simulink model "Model_v2"  (R2016b)
settings: Solver=VariableStepAuto  StartTime=0.0  StopTime=2  MaxStep=0.01  RelTol=1e-3
InitFcn:
  | start
values from neighbouring files (symbols this model uses):
  A = [0 0 1 ... (first row only)    [matrix_set.m]
  B = [0 ... (first row only)    [matrix_set.m]
  K = lqr(A,B,QQ,RR)    [matrix_set.m]
  Psi0 = pi/12    (= 0.261799387799)    [start_config.m]
  Psi_d0 = 0    [start_config.m]
  R = 0.0275    [variables_set.m]
  Theta_d0 = 0    [start_config.m]
  Umax = 8.2    [variables_set.m]
libraries: vrlib x4, simulink_extras x3
settings Model: PauseTimes=1  SnapshotBufferSize=8000  Creator=danii  LastModifiedBy=danii
settings SolverCC: ZeroCrossAlgorithm=Adaptive
settings ConfigComp: PSAutoStubLUT=on

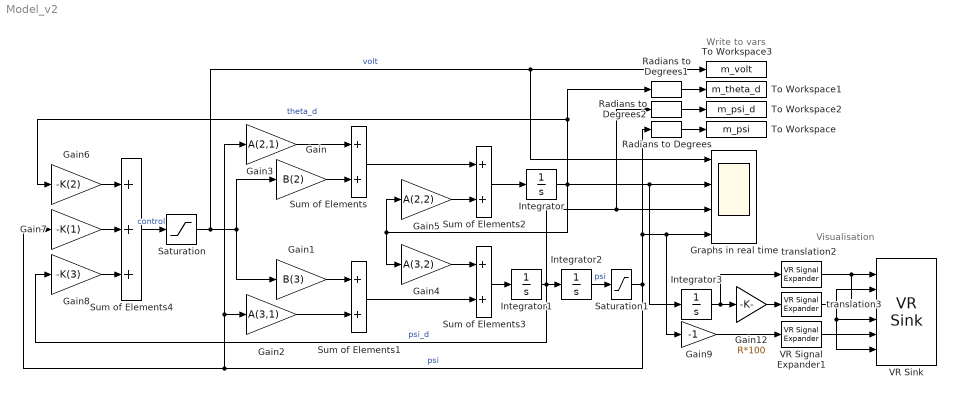
== system Model_v2 ==
  note: Visualisation
  note: Write to vars
  Gain : Gain  Gain=B(2)
  Gain1 : Gain  Gain=B(3)
  Gain12 : Gain  Gain=R*100
  Gain2 : Gain  Gain=A(3,1)
  Gain3 : Gain  Gain=A(2,1)
  Gain4 : Gain  Gain=A(3,2)
  Gain5 : Gain  Gain=A(2,2)
  Gain6 : Gain  Gain=-K(2)
  Gain7 : Gain  Gain=-K(1)
  Gain8 : Gain  Gain=-K(3)
  Gain9 : Gain  Gain=-1
  Graphs in real time : Scope  NumInputPorts=4
  Integrator : Integrator  InitialCondition=Theta_d0
  Integrator1 : Integrator  InitialCondition=Psi_d0
  Integrator2 : Integrator  InitialCondition=Psi0
  Integrator3 : Integrator  InitialCondition=Theta_d0
  Radians to Degrees : simulink_extras/Transformations/Radians to Degrees
  Radians to Degrees1 : simulink_extras/Transformations/Radians to Degrees
  Radians to Degrees2 : simulink_extras/Transformations/Radians to Degrees
  Saturation : Saturate  UpperLimit=Umax  LowerLimit=-Umax
  Saturation1 : Saturate  UpperLimit=pi/180*95  LowerLimit=-pi/180*95
  Sum of Elements{,1..3} (4 alike) : Sum  Inputs=2
  Sum of Elements4 : Sum  Inputs=3
  To Workspace : ToWorkspace  VariableName=m_psi  SampleTime=-1
  To Workspace1 : ToWorkspace  VariableName=m_theta_d  SampleTime=-1
  To Workspace2 : ToWorkspace  VariableName=m_psi_d  SampleTime=-1
  To Workspace3 : ToWorkspace  VariableName=m_volt  SampleTime=-1
  VR Signal Expander1 : vrlib/VR Signal Expander  outwidth=4  outidx=[4]
  VR Sink : vrlib/VR Sink  InstantiateOnLoad=on  SampleTime=0.005  ViewEnable=on  RemoteChange=off  RemoteView=off  FieldsWritten=wheel_1.rotation.4.1.1.double#wheel_1.translation.3.1.1.double#wheel_2.rotation.4.1.1.double#wheel_2.translation.3.1.1.double#body.rotation.4.1.1.double#body.translation.3.1.1.double  WorldFileName=Model.wrl  AutoView=off  VideoDimensions=[]  AllowVariableSize=off  FigureProperties="{'Position', 'Name', 'Viewpoint', 'CameraBound', 'CameraDirection', 'CameraPosition', 'CameraUpVector', 'ZoomFactor', 'Antialiasing', 'Headlight', 'Lighting', 'NavPanel', 'Sound', 'StatusBar', 'Stereo3D', 'Stereo3DCameraOffset', 'Stereo3DHIT', 'ToolBar', 'Textures', 'Transparency', 'Triad', 'Wireframe', 'NavZones', 'NavMode', 'NavSpeed', 'CaptureFileFormat', 'CaptureFileName', 'Record2DCompressMethod', 'Record2DCompressQuality', 'Record2D', 'Record2DFileName', 'Record2DFPS'; [5.0000000000000000e+00   9.2000000000000000e+01   5.7600000000000000e+02   3.5000000000000000e+02], '', '2', 'on', [0.0000000000000000e+00   0.0000000000000000e+00  -1.0000000000000000e+00], [0.0000000000000000e+00   0.0000000000000000e+00   0.0000000000000000e+00], [0.0000000000000000e+00   1.0000000000000000e+00   0.0000000000000000e+00], [1.0000000000000000e+00], 'on', 'on', 'on', 'halfbar', 'on', 'on', 'off', [1.0000000149011612e-01], [0.0000000000000000e+00], 'on', 'on', 'on', 'none', 'off', 'off', 'fly', 'normal', 'tif', '%f_anim_%n.tif', 'auto', [7.5000000000000000e+01], 'off', '%f_anim_%n.avi', 'auto'}"
  translation2 : vrlib/VR Signal Expander  outwidth=4  outidx=[1]
  translation3 : vrlib/VR Signal Expander  outwidth=3  outidx=[1]
  wires:
  Saturation/1 -> Graphs in real time/1, To Workspace3/1, Gain1/1, Gain/1  "volt"
  Gain/1 -> Sum of Elements/2
  Gain1/1 -> Sum of Elements1/1
  Gain2/1 -> Sum of Elements1/2
  Gain3/1 -> Sum of Elements/1
  Sum of Elements/1 -> Sum of Elements2/1
  Sum of Elements1/1 -> Sum of Elements3/2
  Gain5/1 -> Sum of Elements2/2
  Gain4/1 -> Sum of Elements3/1
  Sum of Elements2/1 -> Integrator/1
  Sum of Elements3/1 -> Integrator1/1
  Integrator/1 -> Gain4/1, Gain5/1, Integrator3/1, Graphs in real time/2, Gain6/1, Radians to Degrees1/1  "theta_d"
  Integrator1/1 -> Integrator2/1, Gain8/1, Radians to Degrees2/1, Graphs in real time/3  "psi_d"
  Sum of Elements4/1 -> Saturation/1  "control"
  Gain7/1 -> Sum of Elements4/2
  Gain8/1 -> Sum of Elements4/3
  Radians to Degrees/1 -> To Workspace/1
  Radians to Degrees2/1 -> To Workspace2/1
  Radians to Degrees1/1 -> To Workspace1/1
  Integrator2/1 -> Saturation1/1  "psi"
  Gain6/1 -> Sum of Elements4/1
  translation2/1 -> VR Sink/3, VR Sink/1
  Gain12/1 -> translation3/1
  translation3/1 -> VR Sink/6, VR Sink/4, VR Sink/2
  VR Signal Expander1/1 -> VR Sink/5
  Gain9/1 -> VR Signal Expander1/1
  Saturation1/1 -> Gain7/1, Gain3/1, Gain2/1, Radians to Degrees/1, Graphs in real time/4, Gain9/1  "psi"
  Integrator3/1 -> Gain12/1, translation2/1
